simulink model "PlantModels"  (R2024a)
settings: Solver=VariableStepAuto  StartTime=0.0  StopTime=10  RelTol=1e-3
model workspace (MAT data in the model file):
  g = Simulink.Parameter
  g.Value = 9.80665
  g.Complexity = 'real'
  g.Dimensions = [1 1]
  g.DataType = 'auto'
  l = Simulink.Parameter
  l.Value = 3.7
  l.Complexity = 'real'
  l.Dimensions = [1 1]
  l.DataType = 'auto'
settings Model: Creator=Riley  LastModifiedBy=Riley
settings DataIOCC: ExternalInput=crane_data.getElement('crane_position'),crane_data.getElement('hoist_speed')  LoadExternalInput=on

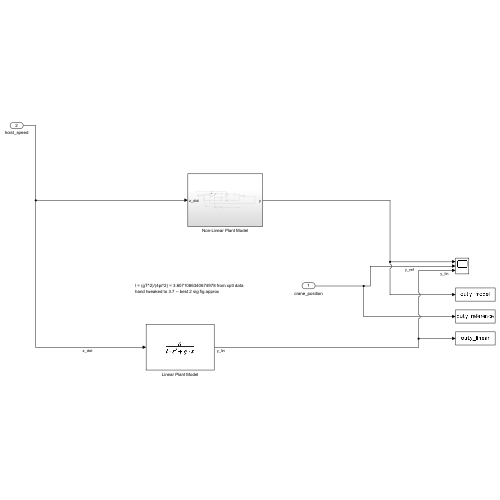
[thumbnail: Simulink's stored preview of the top-level diagram]
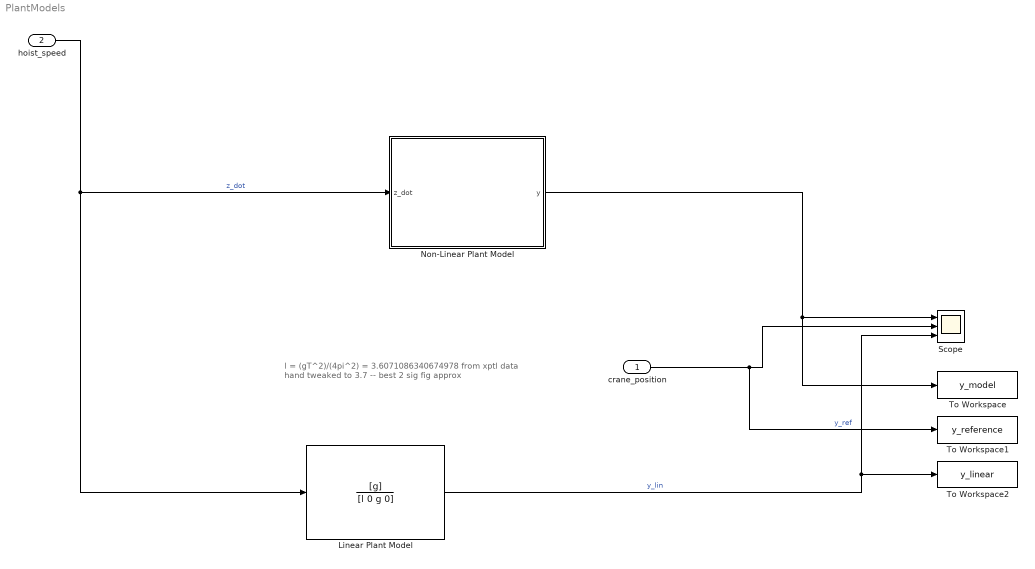
== system PlantModels ==
  note: l = (gT^2)/(4pi^2) = 3.6071086340674978 from xptl data
      | hand tweaked to 3.7 -- best 2 sig fig approx
  crane_position : Inport
  hoist_speed : Inport  Port=2
  Linear Plant Model : TransferFcn  Numerator=[g]  Denominator=[l 0 g 0]
  Non-Linear Plant Model : Subsystem
  Scope : Scope  NumInputPorts=3
  To Workspace : ToWorkspace  VariableName=y_model  SaveFormat=Timeseries  SampleTime=-1
  To Workspace1 : ToWorkspace  VariableName=y_reference  SaveFormat=Timeseries  SampleTime=-1
  To Workspace2 : ToWorkspace  VariableName=y_linear  SaveFormat=Timeseries  SampleTime=-1
  wires:
  hoist_speed/1 -> Non-Linear Plant Model/1(z_dot), Linear Plant Model/1  "z_dot"
  crane_position/1 -> To Workspace1/1, Scope/2  "y_ref"
  Linear Plant Model/1 -> Scope/3, To Workspace2/1  "y_lin"
  Non-Linear Plant Model/1(y) -> Scope/1, To Workspace/1

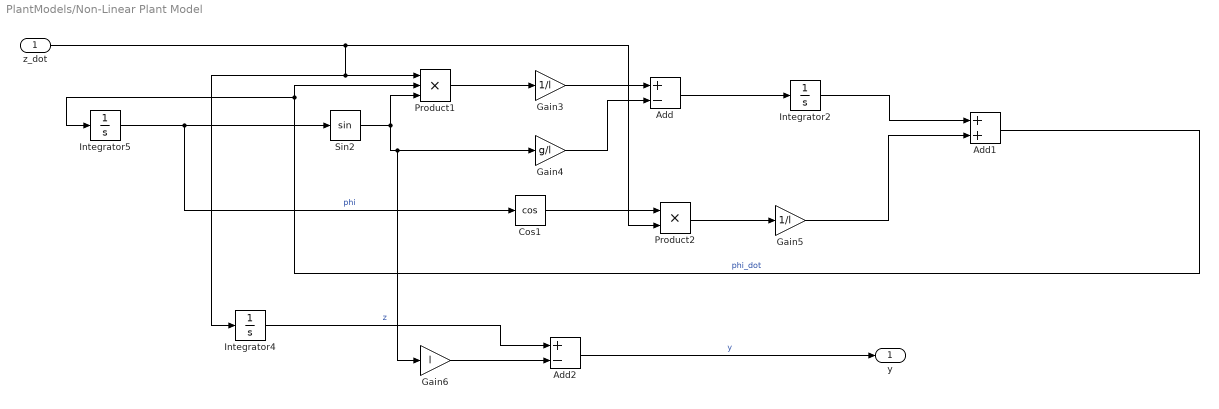
== system PlantModels/Non-Linear Plant Model ==
  z_dot : Inport
  Add : Sum  Inputs=+-
  Add1 : Sum
  Add2 : Sum  Inputs=+-
  Cos1 : Trigonometry  Operator=cos
  Gain3 : Gain  Gain=1/l
  Gain4 : Gain  Gain=g/l
  Gain5 : Gain  Gain=1/l
  Gain6 : Gain  Gain=l
  Integrator2 : Integrator
  Integrator4 : Integrator
  Integrator5 : Integrator
  Product1 : Product  Inputs=3
  Product2 : Product
  Sin2 : Trigonometry
  y : Outport
  wires:
  z_dot/1 -> Integrator4/1, Product1/1, Product2/2
  Sin2/1 -> Gain4/1, Gain6/1, Product1/3
  Product1/1 -> Gain3/1
  Add1/1 -> Product1/2, Integrator5/1  "phi_dot"
  Gain3/1 -> Add/1
  Integrator5/1 -> Cos1/1, Sin2/1  "phi"
  Integrator2/1 -> Add1/1
  Add/1 -> Integrator2/1
  Cos1/1 -> Product2/1
  Product2/1 -> Gain5/1
  Gain4/1 -> Add/2
  Gain5/1 -> Add1/2
  Gain6/1 -> Add2/2
  Integrator4/1 -> Add2/1  "z"
  Add2/1 -> y/1  "y"
